simulink model "discrete_time_vs"  (R2020b)
settings: Solver=ode45  StartTime=0.0  StopTime=10.0  MaxStep=0.5e-3  RelTol=1e-6
values from neighbouring files (symbols this model uses):
  Ts = 0.1    [init.m]
  vMax = 1    [init.m]
  wMax = deg2rad(60)    [init.m]
settings Model: Creator=marco  LastModifiedBy=marco

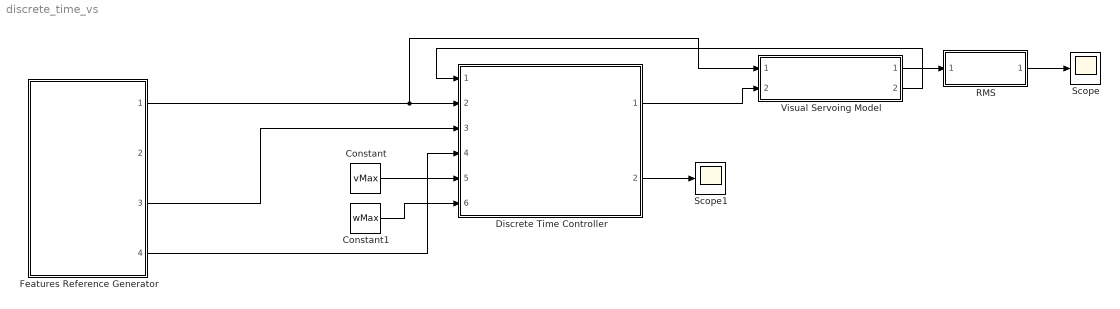
== system discrete_time_vs ==
  Constant : Constant  Value=vMax
  Constant1 : Constant  Value=wMax
  Discrete Time Controller : Subsystem  ReferencedSubsystem=DiscreteTimeController  Ts=Ts  forward_action_enabled=false  use_lambda_const=off  lambdaT_const=.2  use_max_analytic_lambda=on  rmse_noise_level=0.002  l_fcn_disabled=on  val_min=0.06  rmse_noise_slope_max=18  rmse_noise_min=0.002
  Features Reference Generator : Subsystem  ReferencedSubsystem=FeaturesReferenceGenerator  C_features_0=C_features_0  C_features_desired=C_features_desired  Cdesired_T_C0=Cdesired_T_C0.double  Ts=Ts  t0=0  tf=3  no_traj=on
  RMS : Subsystem  ReferencedSubsystem=RMS
  Scope : Scope
  Scope1 : Scope
  Visual Servoing Model : Subsystem  ReferencedSubsystem=Features_System  s0=s0  noise_perc=0.005  noise_sample_time=0.1
  wires:
  Visual Servoing Model/1 -> RMS/1
  RMS/1 -> Scope/1
  Features Reference Generator/1 -> Visual Servoing Model/1, Discrete Time Controller/2
  Features Reference Generator/3 -> Discrete Time Controller/3
  Features Reference Generator/4 -> Discrete Time Controller/4
  Discrete Time Controller/1 -> Visual Servoing Model/2
  Discrete Time Controller/2 -> Scope1/1
  Visual Servoing Model/2 -> Discrete Time Controller/1
  Constant/1 -> Discrete Time Controller/5
  Constant1/1 -> Discrete Time Controller/6
